simulink model "plant"  (R2023b)
settings: Solver=VariableStepAuto  StartTime=0.0  StopTime=10.0  RelTol=1e-3
values from neighbouring files (symbols this model uses):
  An = T*A*inv(T)    [canon_normal.m]
  Bn = T*B    [canon_normal.m]
undefined symbols (not defined in the file or in its folder): g, K, phi, psi
settings Model: Creator=edmli  LastModifiedBy=edmli

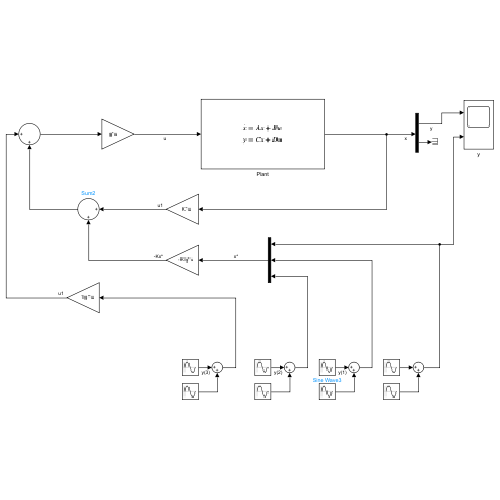
[thumbnail: Simulink's stored preview of the top-level diagram]
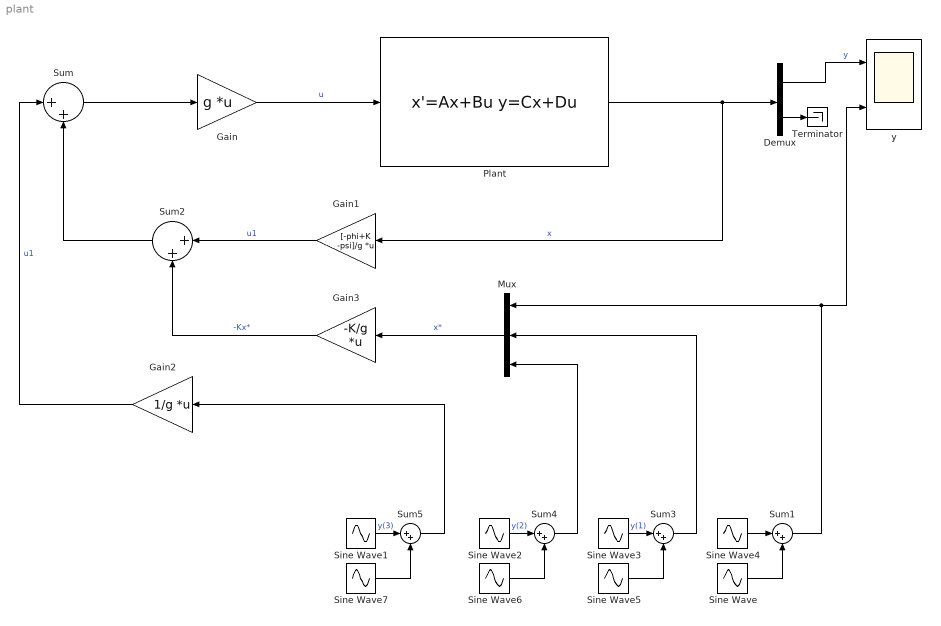
== system plant ==
  Demux : Demux  Outputs=[1 3]
  Gain : Gain  Gain=g  Multiplication=Matrix(K*u)
  Gain1 : Gain  Gain=[-phi+K -psi]/g  Multiplication=Matrix(K*u)
  Gain2 : Gain  Gain=1/g  Multiplication=Matrix(K*u)
  Gain3 : Gain  Gain=-K/g  Multiplication=Matrix(K*u)
  Mux : Mux  Inputs=3
  Plant : StateSpace  A=An  B=Bn  C=eye(4)  D=[0;0;0;0]  InitialCondition=[1;0;0;0]
  Sine Wave : Sin  SampleTime=0
  Sine Wave1 : Sin  Amplitude=250  Frequency=5  Phase=1.5*pi  Samples=100  SampleTime=0
  Sine Wave2 : Sin  Amplitude=50  Frequency=5  Phase=pi  Samples=100  SampleTime=0
  Sine Wave3 : Sin  Amplitude=10  Frequency=5  Phase=pi/2  Samples=100  SampleTime=0
  Sine Wave4 : Sin  Amplitude=2  Frequency=5  Samples=100  SampleTime=0
  Sine Wave5 : Sin  Phase=0.5*pi  SampleTime=0
  Sine Wave6 : Sin  Phase=pi  SampleTime=0
  Sine Wave7 : Sin  Phase=1.5*pi  SampleTime=0
  Sum{,1..5} (6 alike) : Sum  Inputs=|++
  Terminator : Terminator
  y : Scope  NumInputPorts=2
  wires:
  Gain/1 -> Plant/1  "u"
  Plant/1 -> Gain1/1, Demux/1  "x"
  Sum/1 -> Gain/1
  Demux/1 -> y/1  "y"
  Demux/2 -> Terminator/1
  Mux/1 -> Gain3/1  "x*"
  Gain1/1 -> Sum2/1  "u1"
  Gain2/1 -> Sum/1  "u1"
  Gain3/1 -> Sum2/2  "-Kx*"
  Sum2/1 -> Sum/2
  Sine Wave/1 -> Sum1/2
  Sine Wave4/1 -> Sum1/1
  Sum1/1 -> Mux/1, y/2
  Sine Wave5/1 -> Sum3/2
  Sine Wave3/1 -> Sum3/1  "y(1)"
  Sum3/1 -> Mux/2
  Sine Wave6/1 -> Sum4/2
  Sine Wave2/1 -> Sum4/1  "y(2)"
  Sum4/1 -> Mux/3
  Sine Wave7/1 -> Sum5/2
  Sine Wave1/1 -> Sum5/1  "y(3)"
  Sum5/1 -> Gain2/1
